simulink model "kalman_final"  (R2021b)
settings: Solver=VariableStepAuto  StartTime=0.0  StopTime=simTime  FixedStep=0.005  RelTol=1e-3
values from neighbouring files (symbols this model uses):
  bias = -0.3*ones(3,1)    [kalman_ex_5.m]    (also in pitch_kalman_bias.m = -0.3; roll_kalman_bias.m = -0.3)
  P = P.Data(:,:,end)    [kalman_ex_5.m]
  Q = diag([100*cov_wx 100*cov_wy 100*cov_wz 0.1*cov_wx 0.1*cov_wy 0.1*cov_wz])    [kalman_ex_5.m]    (also in pitch_kalman.m = cov_wy; pitch_kalman_bias.m = diag([10000*cov_wy cov_wy]); roll_kalman.m = cov_wx; roll_kalman_bias.m = diag([10000*cov_wx cov_wx]))
  R = 100*R    [kalman_ex_5.m]    (also in pitch_kalman.m = 10*cov_pitch_acel; pitch_kalman_bias.m = 10*cov_pitch_acel; roll_kalman.m = 10*cov_roll_acel; roll_kalman_bias.m = 10*cov_roll_acel)
  var_R = 1    [kalman_ex_5.m]
  x_0 = [0;0; -9.81; -0.3; -0.3; -0.3]    [kalman_ex_5.m]
settings Model: Creator=sasas  LastModifiedBy=p28ma
settings SolverCC: AlgebraicLoopSolver=TrustRegion
settings DebuggingCC: SFMachineParentedDataDiag=warning

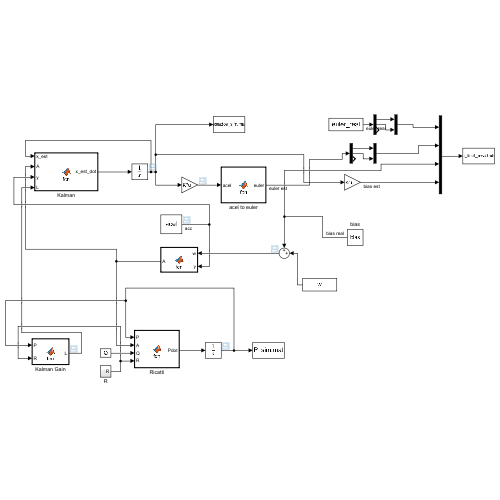
[thumbnail: Simulink's stored preview of the top-level diagram]
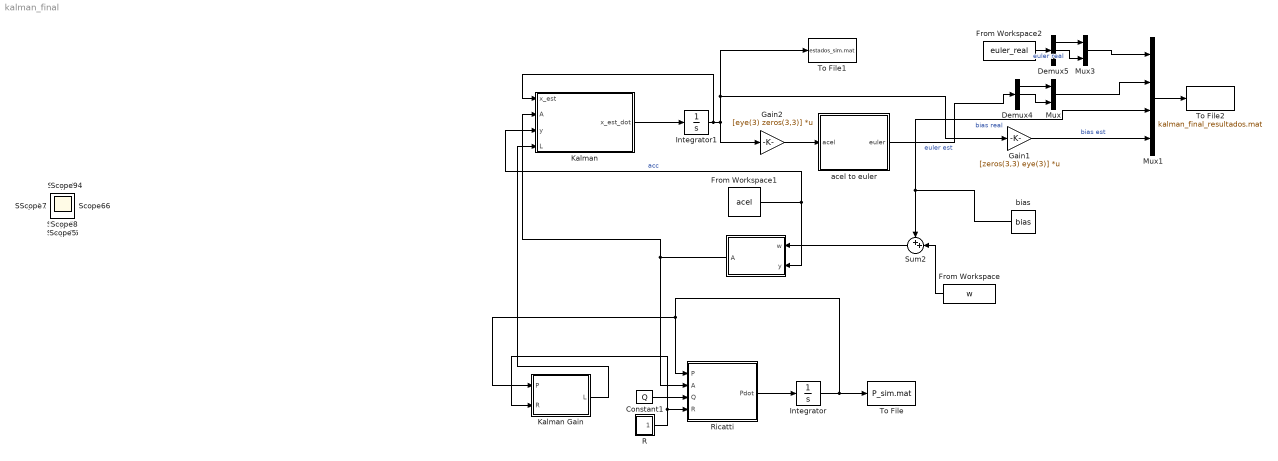
== system kalman_final ==
  " " : MATLAB Function  TreatAsAtomicUnit=on
  Constant1 : Constant  Value=Q
  Demux4 : Demux  Outputs=3
  Demux5 : Demux  Outputs=3
  From Workspace : FromWorkspace  VariableName=w  SampleTime=-1
  From Workspace1 : FromWorkspace  VariableName=acel  SampleTime=-1
  From Workspace2 : FromWorkspace  VariableName=euler_real
  Gain1 : Gain  Gain=[zeros(3,3) eye(3)]  Multiplication=Matrix(K*u)
  Gain2 : Gain  Gain=[eye(3) zeros(3,3)]  Multiplication=Matrix(K*u)
  Integrator : Integrator  InitialCondition=P
  Integrator1 : Integrator  InitialCondition=x_0
  Kalman : MATLAB Function  TreatAsAtomicUnit=on
  Kalman Gain : MATLAB Function  TreatAsAtomicUnit=on
  Mux : Mux  Inputs=2
  Mux1 : Mux
  Mux3 : Mux  Inputs=2
  R : Subsystem
  Ricatti : MATLAB Function  TreatAsAtomicUnit=on
  Sum2 : Sum  Inputs=++|
  To File : ToFile  Filename=P_sim.mat  MatrixName=P_sim  SaveFormat=Timeseries
  To File1 : ToFile  Filename=estados_sim.mat  MatrixName=estados_sim  SaveFormat=Timeseries
  To File2 : ToFile  Filename=kalman_final_resultados.mat  MatrixName=kalman_final_resultados  SaveFormat=Timeseries
  acel to euler : MATLAB Function  TreatAsAtomicUnit=on
  bias : Constant  Value=bias  VectorParams1D=off
  Scope{,1..16} (17 alike) : Scope
  wires:
  Constant1/1 -> Ricatti/3(Q)
  Ricatti/1(Pdot) -> Integrator/1
  Integrator/1 -> To File/1, Ricatti/1(P), Kalman Gain/1(P)
  Gain2/1 -> acel to euler/1(acel)
  bias/1 -> Mux1/3, Sum2/1  "bias real"
  Sum2/1 -> " "/1(w)
  Integrator1/1 -> Kalman/1(x_est), Gain1/1, To File1/1, Gain2/1
  acel to euler/1(euler) -> Demux4/1  "euler est"
  R/1(R) -> Kalman Gain/2(R), Ricatti/4(R)
  From Workspace1/1 -> " "/2(y), Kalman/3(y)  "acc"
  From Workspace/1 -> Sum2/2
  " "/1(A) -> Kalman/2(A), Ricatti/2(A)
  Kalman/1(x_est_dot) -> Integrator1/1
  Kalman Gain/1(L) -> Kalman/4(L)
  Demux4/1 -> Mux/1
  Demux4/2 -> Mux/2
  From Workspace2/1 -> Demux5/1  "euler real"
  Demux5/1 -> Mux3/1
  Demux5/2 -> Mux3/2
  Mux3/1 -> Mux1/1
  Mux/1 -> Mux1/2
  Gain1/1 -> Mux1/4  "bias est"
  Mux1/1 -> To File2/1

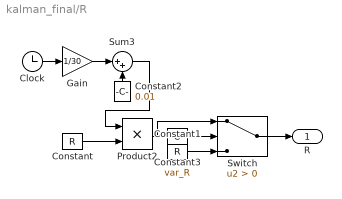
== system kalman_final/R ==
  Clock : Clock
  Constant : Constant  Value=R
  Constant1 : Constant  Value=R
  Constant2 : Constant  Value=0.01
  Constant3 : Constant  Value=var_R
  Gain : Gain  Gain=1/30
  Product2 : Product
  Sum3 : Sum  Inputs=|++
  Switch : Switch  Criteria=u2 > Threshold
  R : Outport
  wires:
  Sum3/1 -> Product2/1
  Gain/1 -> Sum3/1
  Constant2/1 -> Sum3/2
  Clock/1 -> Gain/1
  Constant/1 -> Product2/2
  Switch/1 -> R/1
  Product2/1 -> Switch/1
  Constant1/1 -> Switch/3
  Constant3/1 -> Switch/2

== matlab function kalman_final/Kalman Gain ==
  data: P input; L output; R input
function L = fcn(P,R)
C = [eye(3) zeros(3,3)];
L = P*C'*inv(R);

== matlab function kalman_final/Ricatti ==
  data: P input; Pdot output; A input; Q input; R input
function Pdot = fcn(P,A,Q,R)
C = [eye(3) zeros(3,3)];

Pdot = A*P+P*A'+Q-P*C'*inv(R)*C*P;

== matlab function kalman_final/Kalman ==
  data: x_est input; A input; y input; x_est_dot output; L input
function x_est_dot = fcn(x_est,A,y,L)
C = [eye(3) zeros(3,3)];
x_est_dot = A*x_est + L*(y-C*x_est);

== matlab function kalman_final/  ==
  data: w input; A output; y input
function A = fcn(w,y)
A = [0 w(3) -w(2) 0 y(3) -y(2);
    -w(3) 0 w(1) -y(3) 0 y(1);
    w(2) -w(1) 0 y(2) -y(1) 0;
    0 0 0 0 0 0;
    0 0 0 0 0 0;
    0 0 0 0 0 0];

== matlab function kalman_final/acel to euler ==
  data: acel input; euler output
function euler = fcn(acel)
euler = zeros(3,1);
euler(1) = atan2(-acel(2),-acel(3));
euler(2) = atan2(acel(1),sqrt(acel(2).^2+acel(3).^2));
euler(3) = 0;
